simulink model "cartesian_waypoints_planner"  (R2020a)
settings: Solver=ode3  StartTime=0.0  StopTime=inf  FixedStep=0.01  RelTol=1e-3
undefined symbols (not defined in the file or in its folder): Header, Pose, TimeFromStart
libraries: robotlib x35, robotmaniplib x2, robotcorelib x1
settings Model: Creator=ROS_PO  LastModifiedBy=difra
settings OptimizationCC: EnhancedBackFolding=on  PassReuseOutputArgsAs=Individual arguments  ZeroExternalMemoryAtStartup=off  ZeroInternalMemoryAtStartup=off  MaxStackSize=64  OptimizeBlockOrder=speed  DifferentSizesBufferReuse=on  OptimizationCustomize=off  EfficientTunableParamExpr=on
settings DebuggingCC: ParameterTunabilityLossMsg=error
settings HardwareCC: ProdBitPerPointer=32  ProdBitPerSizeT=32  ProdBitPerPtrDiffT=32  ProdLargestAtomicFloat=None  ProdIntDivRoundTo=Undefined  ProdEndianess=Unspecified  ProdWordSize=32  ProdHWDeviceType=Generic->Unspecified (assume 32-bit Generic)
settings RTWCC: SystemTargetFile=ert.tlc  HardwareBoard=Robot Operating System (ROS)  TemplateMakefile=ert_default_tmf  GenerateReport=on  Toolchain=Catkin  IncludeHyperlinkInReport=on  LaunchReport=on  TargetLang=C++  GenerateTraceInfo=on  GenerateTraceReport=on  GenerateTraceReportSl=on  GenerateTraceReportSf=on  GenerateTraceReportEml=on
settings CodeAppCC: ForceParamTrailComments=on  IgnoreCustomStorageClasses=off  OperatorAnnotations=on  SimulinkDataObjDesc=on  SFDataObjDesc=on  InsertBlockDesc=on
settings ERTTargetCC: SupportContinuousTime=on  SupportVariableSizeSignals=on

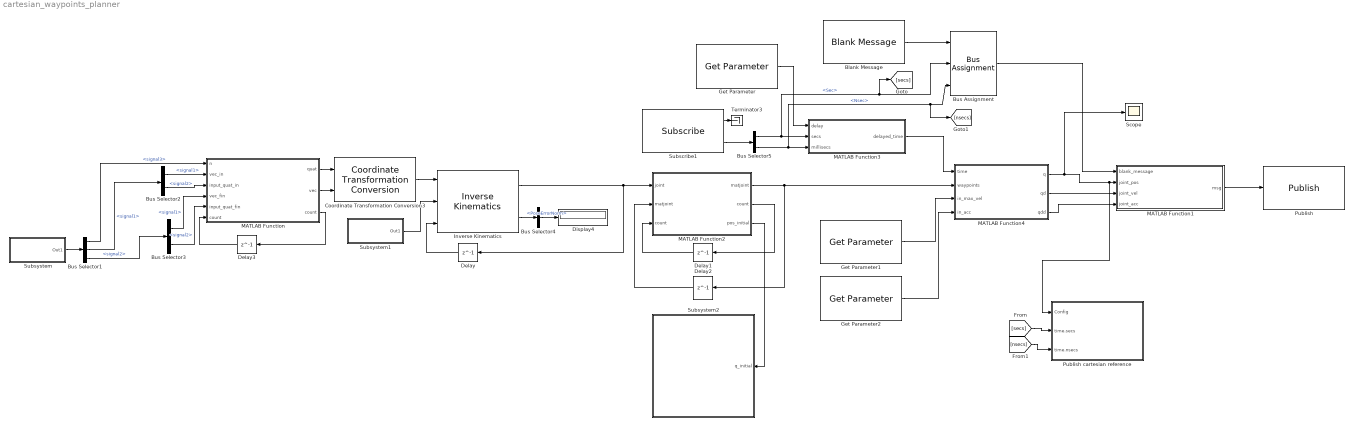
== system cartesian_waypoints_planner ==
  Blank Message : robotlib/Blank Message  messageClass=Message  entityType=trajectory_msgs/JointTrajectoryPoint  messageType=trajectory_msgs/JointTrajectoryPoint  SampleTime=-1
  Bus Assignment : BusAssignment  AssignedSignals=TimeFromStart.Sec,TimeFromStart.Nsec
  Bus Selector1 : BusSelector  OutputSignals=signal3,signal1,signal2
  Bus Selector2 : BusSelector  OutputSignals=signal1,signal2
  Bus Selector3 : BusSelector  OutputSignals=signal1,signal2
  Bus Selector4 : BusSelector  OutputSignals=PoseErrorNorm
  Bus Selector5 : BusSelector  OutputSignals=Clock_.Sec,Clock_.Nsec
  Coordinate Transformation Conversion3 : robotcorelib/Coordinate Transformation Conversion  InputRepresentation=Quaternion  InputEulerSequence=ZYX  ShowTrVecInputPort=on  OutputRepresentation=Homogeneous Transformation  OutputEulerSequence=ZYX  ShowTrVecOutputPort=on  SimulateUsing=Interpreted execution
      settings: SourceProductBaseCode=NV,RO,RR
  Delay : Delay  DelayLength=1  InitialCondition=zeros(6, 1, 1)
  Delay1 : Delay  DelayLength=1  InitialCondition=1
  Delay2 : Delay  DelayLength=1  InitialCondition=zeros(6, 20)
  Delay3 : Delay  DelayLength=1  InitialCondition=1
  Display4 : Display
  Get Parameter : robotlib/Get Parameter  ParameterSource=Specify your own  ParameterName=/start_delay  ParameterType=double  ParameterMaxArrayLength=16  ParameterInitialValue=10  SampleTime=-1  ShowErrorCodeOutput=off  ModelName=cartesian_waypoints_planner  BlockId=ParamGet_cartesian_waypoints_planner_378
      settings: SourceProductBaseCode=RR
  Get Parameter1 : robotlib/Get Parameter  ParameterSource=Specify your own  ParameterName=/max_ang_vel  ParameterType=double  ParameterMaxArrayLength=16  ParameterInitialValue=1  SampleTime=-1  ShowErrorCodeOutput=off  ModelName=cartesian_waypoints_planner  BlockId=ParamGet_cartesian_waypoints_planner_379
      settings: SourceProductBaseCode=RR
  Get Parameter2 : robotlib/Get Parameter  ParameterSource=Specify your own  ParameterName=/max_ang_acc  ParameterType=double  ParameterMaxArrayLength=16  ParameterInitialValue=0.5  SampleTime=-1  ShowErrorCodeOutput=off  ModelName=cartesian_waypoints_planner  BlockId=ParamGet_cartesian_waypoints_planner_380
      settings: SourceProductBaseCode=RR
  Inverse Kinematics : robotmaniplib/Inverse Kinematics  RigidBodyTree=robot  EndEffector=edo_link_ee  ShowInfo=on  SolverName=BFGS Gradient Projection  EnforceJointLimits=on  MaxIterations=1500  MaxTime=10  GradientTolerance=1e-7  SolutionTolerance=1e-6  StepTolerance=1e-14  ErrorChangeTolerance=1e-12  UseErrorDamping=on  DampingBias=0.0025  SimulateUsing=Interpreted execution
  MATLAB Function : MATLAB Function  TreatAsAtomicUnit=on
  MATLAB Function1 : MATLAB Function  TreatAsAtomicUnit=on
  MATLAB Function2 : MATLAB Function  TreatAsAtomicUnit=on
  MATLAB Function3 : MATLAB Function  TreatAsAtomicUnit=on
  MATLAB Function4 : MATLAB Function  TreatAsAtomicUnit=on
  Publish : robotlib/Publish  topicSource=Select from ROS network  topic=/joint_trajectory  messageType=trajectory_msgs/JointTrajectoryPoint  messageQueueLength=1
      link override SinkBlock: ROSTopic=/joint_trajectory  ROSMessageType=trajectory_msgs/JointTrajectoryPoint  SLBusName=SL_Bus_joint_trajectory_planner_JointTrajectoryPoint_y0wep  ModelName=joint_trajectory_planner  BlockId=Pub_joint_trajectory_planner_5
  Publish cartesian reference : Subsystem
  Scope : Scope
  Subscribe1 : robotlib/Subscribe  topicSource=Specify your own  topic=/clock  messageType=rosgraph_msgs/Clock  sampleTime=-1  messageQueueLength=1
  Subsystem : Subsystem
  Subsystem1 : Subsystem
  Subsystem2 : Subsystem
  Terminator3 : Terminator
  wires:
  Subsystem1/1(Out1) -> Inverse Kinematics/2
  Bus Selector4/1 -> Display4/1  "<PoseErrorNorm>"
  Inverse Kinematics/1 -> Delay/1, MATLAB Function2/1(joint)
  Inverse Kinematics/2 -> Bus Selector4/1
  Delay/1 -> Inverse Kinematics/3
  Subsystem/1(Out1) -> Bus Selector1/1
  Delay1/1 -> MATLAB Function2/3("count ")
  MATLAB Function2/2(count) -> Delay1/1
  Delay2/1 -> MATLAB Function2/2("matjoint ")
  MATLAB Function/3(count) -> Delay3/1
  Delay3/1 -> MATLAB Function/6("count ")
  MATLAB Function/1(quat) -> Coordinate Transformation Conversion3/1
  MATLAB Function/2(vec) -> Coordinate Transformation Conversion3/2
  Coordinate Transformation Conversion3/1 -> Inverse Kinematics/1
  Bus Selector2/1 -> MATLAB Function/2(vec_in)  "<signal1>"
  Bus Selector2/2 -> MATLAB Function/3(input_quat_in)  "<signal2>"
  Bus Selector3/1 -> MATLAB Function/4(vec_fin)  "<signal1>"
  Bus Selector3/2 -> MATLAB Function/5(input_quat_fin)  "<signal2>"
  Bus Selector1/3 -> Bus Selector3/1  "<signal2>"
  Bus Selector1/2 -> Bus Selector2/1  "<signal1>"
  Bus Selector1/1 -> MATLAB Function/1(n)  "<signal3>"
  MATLAB Function2/3(pos_initial) -> Subsystem2/1(q_initial)
  Subscribe1/1 -> Terminator3/1
  Get Parameter1/1 -> MATLAB Function4/3(in_max_vel)
  Bus Selector5/1 -> [secs], Bus Assignment/2, MATLAB Function3/2(secs)  "<Sec>"
  Bus Selector5/2 -> [nsecs], Bus Assignment/3, MATLAB Function3/3(millisecs)  "<Nsec>"
  Get Parameter/1 -> MATLAB Function3/1(delay)
  Subscribe1/2 -> Bus Selector5/1
  Get Parameter2/1 -> MATLAB Function4/4(in_acc)
  MATLAB Function4/2(qd) -> MATLAB Function1/3(joint_vel)
  MATLAB Function4/1(q) -> Scope/1, Publish cartesian reference/1(Config), MATLAB Function1/2(joint_pos)
  Blank Message/1 -> Bus Assignment/1
  MATLAB Function1/1(msg) -> Publish/1
  MATLAB Function4/3(qdd) -> MATLAB Function1/4(joint_acc)
  Bus Assignment/1 -> MATLAB Function1/1(blank_message)
  [nsecs] -> Publish cartesian reference/3(time.nsecs)
  [secs] -> Publish cartesian reference/2(time.secs)
  MATLAB Function3/1(delayed_time) -> MATLAB Function4/1(time)
  MATLAB Function2/1(matjoint) -> MATLAB Function4/2(waypoints), Delay2/1

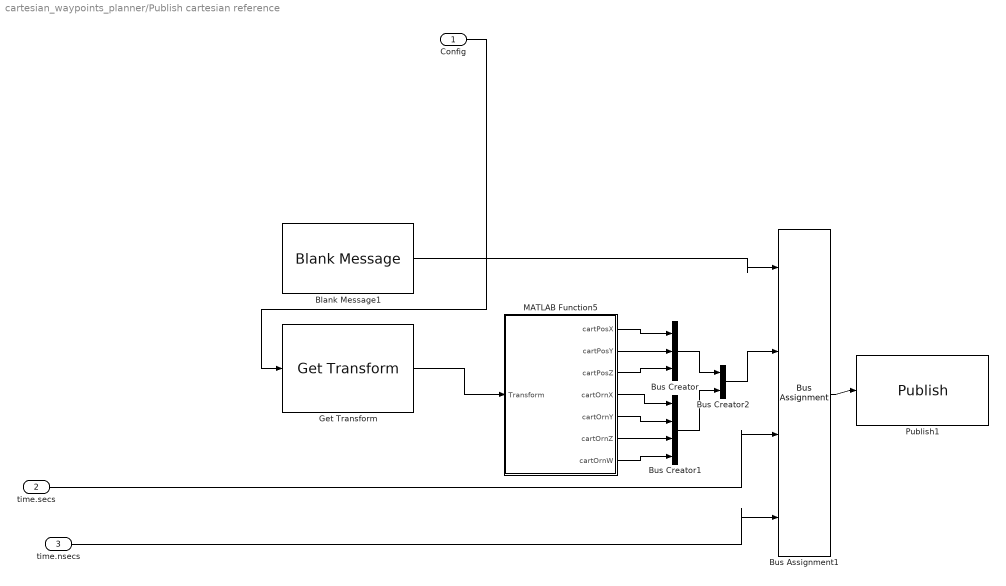
== system cartesian_waypoints_planner/Publish cartesian reference ==
  Config : Inport
  time.secs : Inport  Port=2
  time.nsecs : Inport  Port=3
  Blank Message1 : robotlib/Blank Message  messageClass=Message  entityType=geometry_msgs/PoseStamped  messageType=geometry_msgs/PoseStamped  SampleTime=inf
  Bus Assignment1 : BusAssignment  AssignedSignals=Pose,Header.Stamp.Sec,Header.Stamp.Nsec
  Bus Creator : BusCreator  Inputs=3
  Bus Creator1 : BusCreator  Inputs=4
  Bus Creator2 : BusCreator  Inputs=2
  Get Transform : robotmaniplib/Get Transform  RigidBodyTree=robot  SourceBody=edo_link_ee  TargetBody=world  SimulateUsing=Interpreted execution
  MATLAB Function5 : MATLAB Function  TreatAsAtomicUnit=on
  Publish1 : robotlib/Publish  topicSource=Specify your own  topic=/cartesian_trajectory  messageType=geometry_msgs/PoseStamped  messageQueueLength=1
  wires:
  Bus Creator1/1 -> Bus Creator2/2
  time.secs/1 -> Bus Assignment1/3
  MATLAB Function5/3(cartPosZ) -> Bus Creator/3
  MATLAB Function5/6(cartOrnZ) -> Bus Creator1/3
  time.nsecs/1 -> Bus Assignment1/4
  MATLAB Function5/5(cartOrnY) -> Bus Creator1/2
  MATLAB Function5/4(cartOrnX) -> Bus Creator1/1
  MATLAB Function5/2(cartPosY) -> Bus Creator/2
  Get Transform/1 -> MATLAB Function5/1(Transform)
  MATLAB Function5/7(cartOrnW) -> Bus Creator1/4
  Config/1 -> Get Transform/1
  Bus Creator/1 -> Bus Creator2/1
  MATLAB Function5/1(cartPosX) -> Bus Creator/1
  Bus Assignment1/1 -> Publish1/1
  Bus Creator2/1 -> Bus Assignment1/2
  Blank Message1/1 -> Bus Assignment1/1

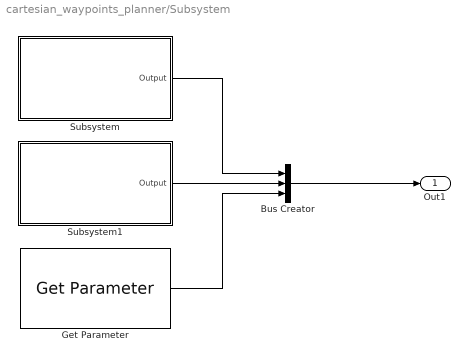
== system cartesian_waypoints_planner/Subsystem ==
  Bus Creator : BusCreator  Inputs=3
  Get Parameter : robotlib/Get Parameter  ParameterSource=Specify your own  ParameterName=/n_points  ParameterType=int32  ParameterMaxArrayLength=16  ParameterInitialValue=3  SampleTime=-1  ShowErrorCodeOutput=off  ModelName=cartesian_waypoints_planner  BlockId=ParamGet_cartesian_waypoints_planner_346
      settings: SourceProductBaseCode=RR
  Subsystem : Subsystem
  Subsystem1 : Subsystem
  Out1 : Outport
  wires:
  Bus Creator/1 -> Out1/1
  Subsystem/1(Output) -> Bus Creator/1
  Get Parameter/1 -> Bus Creator/3
  Subsystem1/1(Output) -> Bus Creator/2

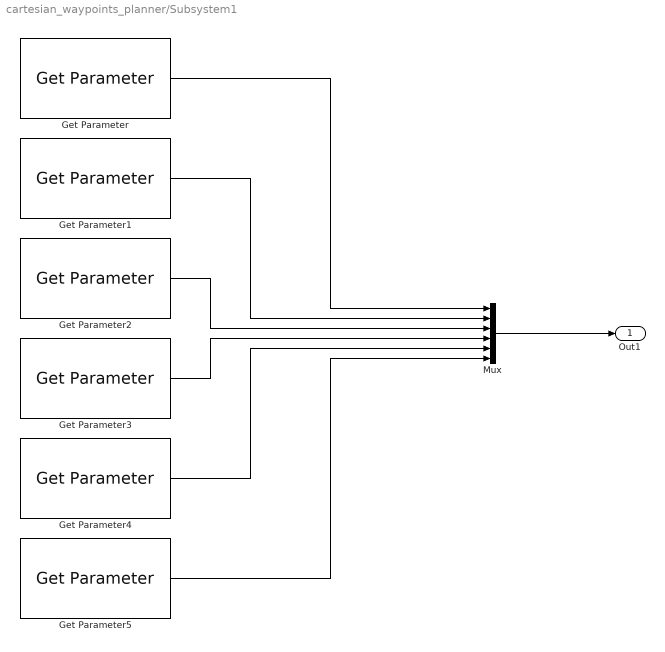
== system cartesian_waypoints_planner/Subsystem1 ==
  Get Parameter : robotlib/Get Parameter  ParameterSource=Specify your own  ParameterName=/weight_ox  ParameterType=double  ParameterMaxArrayLength=16  ParameterInitialValue=0  SampleTime=-1  ShowErrorCodeOutput=off  ModelName=cartesian_waypoints_planner  BlockId=ParamGet_cartesian_waypoints_planner_312
      settings: SourceProductBaseCode=RR
  Get Parameter1 : robotlib/Get Parameter  ParameterSource=Specify your own  ParameterName=/weight_oy  ParameterType=double  ParameterMaxArrayLength=16  ParameterInitialValue=0  SampleTime=-1  ShowErrorCodeOutput=off  ModelName=cartesian_waypoints_planner  BlockId=ParamGet_cartesian_waypoints_planner_313
      settings: SourceProductBaseCode=RR
  Get Parameter2 : robotlib/Get Parameter  ParameterSource=Specify your own  ParameterName=/weight_oz  ParameterType=double  ParameterMaxArrayLength=16  ParameterInitialValue=0  SampleTime=-1  ShowErrorCodeOutput=off  ModelName=cartesian_waypoints_planner  BlockId=ParamGet_cartesian_waypoints_planner_314
      settings: SourceProductBaseCode=RR
  Get Parameter3 : robotlib/Get Parameter  ParameterSource=Specify your own  ParameterName=/weight_px  ParameterType=double  ParameterMaxArrayLength=16  ParameterInitialValue=1  SampleTime=-1  ShowErrorCodeOutput=off  ModelName=cartesian_waypoints_planner  BlockId=ParamGet_cartesian_waypoints_planner_315
      settings: SourceProductBaseCode=RR
  Get Parameter4 : robotlib/Get Parameter  ParameterSource=Specify your own  ParameterName=/weight_py  ParameterType=double  ParameterMaxArrayLength=16  ParameterInitialValue=1  SampleTime=-1  ShowErrorCodeOutput=off  ModelName=cartesian_waypoints_planner  BlockId=ParamGet_cartesian_waypoints_planner_316
      settings: SourceProductBaseCode=RR
  Get Parameter5 : robotlib/Get Parameter  ParameterSource=Specify your own  ParameterName=/weight_pz  ParameterType=double  ParameterMaxArrayLength=16  ParameterInitialValue=1  SampleTime=-1  ShowErrorCodeOutput=off  ModelName=cartesian_waypoints_planner  BlockId=ParamGet_cartesian_waypoints_planner_317
      settings: SourceProductBaseCode=RR
  Mux : Mux  Inputs=6
  Out1 : Outport
  wires:
  Mux/1 -> Out1/1
  Get Parameter/1 -> Mux/1
  Get Parameter1/1 -> Mux/2
  Get Parameter5/1 -> Mux/6
  Get Parameter4/1 -> Mux/5
  Get Parameter3/1 -> Mux/4
  Get Parameter2/1 -> Mux/3

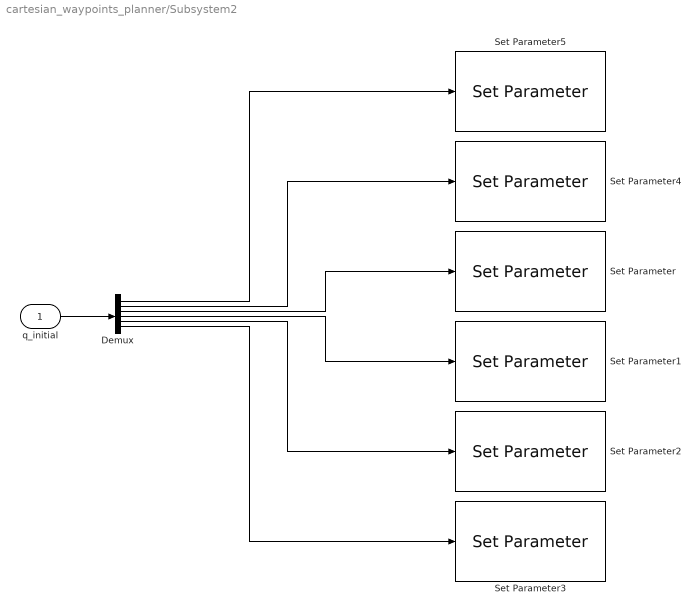
== system cartesian_waypoints_planner/Subsystem2 ==
  q_initial : Inport
  Demux : Demux  Outputs=6
  Set Parameter : robotlib/Set Parameter  ParameterSource=Specify your own  ParameterName=/q3_initial  ParameterType=double  ModelName=cartesian_waypoints_planner  BlockId=ParamSet_cartesian_waypoints_planner_364
      settings: SourceProductBaseCode=RR
  Set Parameter1 : robotlib/Set Parameter  ParameterSource=Specify your own  ParameterName=/q4_initial  ParameterType=double  ModelName=cartesian_waypoints_planner  BlockId=ParamSet_cartesian_waypoints_planner_365
      settings: SourceProductBaseCode=RR
  Set Parameter2 : robotlib/Set Parameter  ParameterSource=Specify your own  ParameterName=/q5_initial  ParameterType=double  ModelName=cartesian_waypoints_planner  BlockId=ParamSet_cartesian_waypoints_planner_366
      settings: SourceProductBaseCode=RR
  Set Parameter3 : robotlib/Set Parameter  ParameterSource=Specify your own  ParameterName=/q6_initial  ParameterType=double  ModelName=cartesian_waypoints_planner  BlockId=ParamSet_cartesian_waypoints_planner_371
      settings: SourceProductBaseCode=RR
  Set Parameter4 : robotlib/Set Parameter  ParameterSource=Specify your own  ParameterName=/q2_initial  ParameterType=double  ModelName=cartesian_waypoints_planner  BlockId=ParamSet_cartesian_waypoints_planner_372
      settings: SourceProductBaseCode=RR
  Set Parameter5 : robotlib/Set Parameter  ParameterSource=Specify your own  ParameterName=/q1_initial  ParameterType=double  ModelName=cartesian_waypoints_planner  BlockId=ParamSet_cartesian_waypoints_planner_373
      settings: SourceProductBaseCode=RR
  wires:
  q_initial/1 -> Demux/1
  Demux/1 -> Set Parameter5/1
  Demux/2 -> Set Parameter4/1
  Demux/3 -> Set Parameter/1
  Demux/4 -> Set Parameter1/1
  Demux/5 -> Set Parameter2/1
  Demux/6 -> Set Parameter3/1

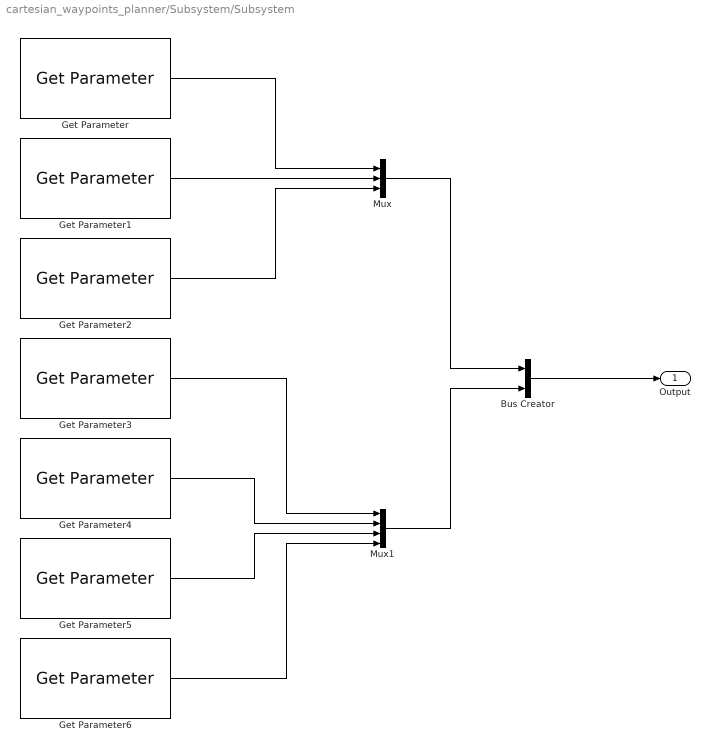
== system cartesian_waypoints_planner/Subsystem/Subsystem ==
  Bus Creator : BusCreator  Inputs=2
  Get Parameter : robotlib/Get Parameter  ParameterSource=Specify your own  ParameterName=/pi_x  ParameterType=double  ParameterMaxArrayLength=16  ParameterInitialValue=0.0  SampleTime=-1  ShowErrorCodeOutput=off  ModelName=cartesian_waypoints_planner  BlockId=ParamGet_cartesian_waypoints_planner_288
      settings: SourceProductBaseCode=RR
  Get Parameter1 : robotlib/Get Parameter  ParameterSource=Specify your own  ParameterName=/pi_y  ParameterType=double  ParameterMaxArrayLength=16  ParameterInitialValue=0.0  SampleTime=-1  ShowErrorCodeOutput=off  ModelName=cartesian_waypoints_planner  BlockId=ParamGet_cartesian_waypoints_planner_289
      settings: SourceProductBaseCode=RR
  Get Parameter2 : robotlib/Get Parameter  ParameterSource=Specify your own  ParameterName=/pi_z  ParameterType=double  ParameterMaxArrayLength=16  ParameterInitialValue=0.99  SampleTime=-1  ShowErrorCodeOutput=off  ModelName=cartesian_waypoints_planner  BlockId=ParamGet_cartesian_waypoints_planner_290
      settings: SourceProductBaseCode=RR
  Get Parameter3 : robotlib/Get Parameter  ParameterSource=Specify your own  ParameterName=/oi_x  ParameterType=double  ParameterMaxArrayLength=16  ParameterInitialValue=0  SampleTime=-1  ShowErrorCodeOutput=off  ModelName=cartesian_waypoints_planner  BlockId=ParamGet_cartesian_waypoints_planner_291
      settings: SourceProductBaseCode=RR
  Get Parameter4 : robotlib/Get Parameter  ParameterSource=Specify your own  ParameterName=/oi_y  ParameterType=double  ParameterMaxArrayLength=16  ParameterInitialValue=0.0  SampleTime=-1  ShowErrorCodeOutput=off  ModelName=cartesian_waypoints_planner  BlockId=ParamGet_cartesian_waypoints_planner_292
      settings: SourceProductBaseCode=RR
  Get Parameter5 : robotlib/Get Parameter  ParameterSource=Specify your own  ParameterName=/oi_z  ParameterType=double  ParameterMaxArrayLength=16  ParameterInitialValue=0.0  SampleTime=-1  ShowErrorCodeOutput=off  ModelName=cartesian_waypoints_planner  BlockId=ParamGet_cartesian_waypoints_planner_293
      settings: SourceProductBaseCode=RR
  Get Parameter6 : robotlib/Get Parameter  ParameterSource=Specify your own  ParameterName=/oi_w  ParameterType=double  ParameterMaxArrayLength=16  ParameterInitialValue=1  SampleTime=-1  ShowErrorCodeOutput=off  ModelName=cartesian_waypoints_planner  BlockId=ParamGet_cartesian_waypoints_planner_294
      settings: SourceProductBaseCode=RR
  Mux : Mux  Inputs=3
  Mux1 : Mux
  Output : Outport
  wires:
  Mux/1 -> Bus Creator/1
  Get Parameter/1 -> Mux/1
  Get Parameter1/1 -> Mux/2
  Get Parameter2/1 -> Mux/3
  Get Parameter3/1 -> Mux1/1
  Get Parameter4/1 -> Mux1/2
  Get Parameter5/1 -> Mux1/3
  Get Parameter6/1 -> Mux1/4
  Mux1/1 -> Bus Creator/2
  Bus Creator/1 -> Output/1

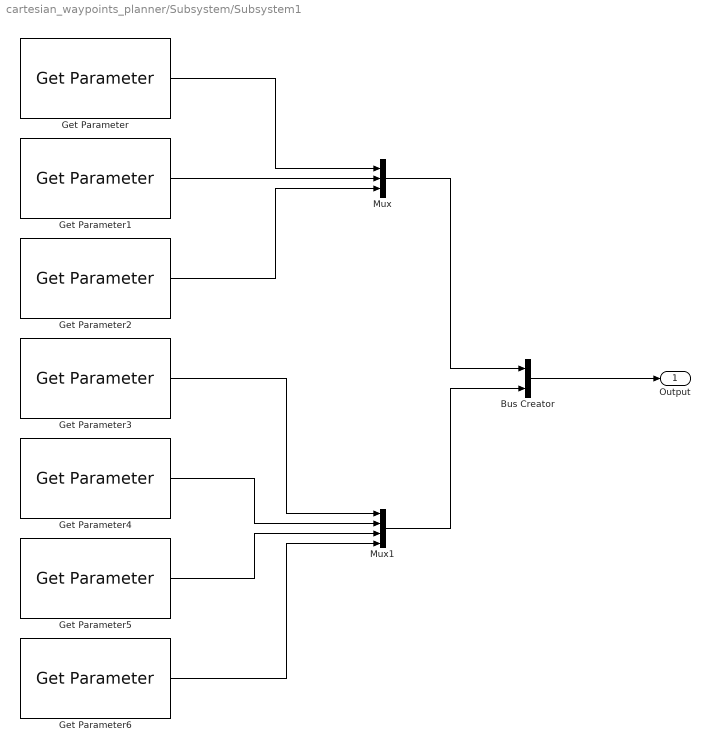
== system cartesian_waypoints_planner/Subsystem/Subsystem1 ==
  Bus Creator : BusCreator  Inputs=2
  Get Parameter : robotlib/Get Parameter  ParameterSource=Specify your own  ParameterName=/pf_x  ParameterType=double  ParameterMaxArrayLength=16  ParameterInitialValue=0.3  SampleTime=-1  ShowErrorCodeOutput=off  ModelName=cartesian_waypoints_planner  BlockId=ParamGet_cartesian_waypoints_planner_300
      settings: SourceProductBaseCode=RR
  Get Parameter1 : robotlib/Get Parameter  ParameterSource=Specify your own  ParameterName=/pf_y  ParameterType=double  ParameterMaxArrayLength=16  ParameterInitialValue=0.3  SampleTime=-1  ShowErrorCodeOutput=off  ModelName=cartesian_waypoints_planner  BlockId=ParamGet_cartesian_waypoints_planner_301
      settings: SourceProductBaseCode=RR
  Get Parameter2 : robotlib/Get Parameter  ParameterSource=Specify your own  ParameterName=/pf_z  ParameterType=double  ParameterMaxArrayLength=16  ParameterInitialValue=0.3  SampleTime=-1  ShowErrorCodeOutput=off  ModelName=cartesian_waypoints_planner  BlockId=ParamGet_cartesian_waypoints_planner_302
      settings: SourceProductBaseCode=RR
  Get Parameter3 : robotlib/Get Parameter  ParameterSource=Specify your own  ParameterName=/of_x  ParameterType=double  ParameterMaxArrayLength=16  ParameterInitialValue=0.39  SampleTime=-1  ShowErrorCodeOutput=off  ModelName=cartesian_waypoints_planner  BlockId=ParamGet_cartesian_waypoints_planner_303
      settings: SourceProductBaseCode=RR
  Get Parameter4 : robotlib/Get Parameter  ParameterSource=Specify your own  ParameterName=/of_y  ParameterType=double  ParameterMaxArrayLength=16  ParameterInitialValue=0.89  SampleTime=-1  ShowErrorCodeOutput=off  ModelName=cartesian_waypoints_planner  BlockId=ParamGet_cartesian_waypoints_planner_304
      settings: SourceProductBaseCode=RR
  Get Parameter5 : robotlib/Get Parameter  ParameterSource=Specify your own  ParameterName=/of_z  ParameterType=double  ParameterMaxArrayLength=16  ParameterInitialValue=0.2  SampleTime=-1  ShowErrorCodeOutput=off  ModelName=cartesian_waypoints_planner  BlockId=ParamGet_cartesian_waypoints_planner_305
      settings: SourceProductBaseCode=RR
  Get Parameter6 : robotlib/Get Parameter  ParameterSource=Specify your own  ParameterName=/of_w  ParameterType=double  ParameterMaxArrayLength=16  ParameterInitialValue=-0.12  SampleTime=-1  ShowErrorCodeOutput=off  ModelName=cartesian_waypoints_planner  BlockId=ParamGet_cartesian_waypoints_planner_306
      settings: SourceProductBaseCode=RR
  Mux : Mux  Inputs=3
  Mux1 : Mux
  Output : Outport
  wires:
  Mux/1 -> Bus Creator/1
  Get Parameter/1 -> Mux/1
  Get Parameter1/1 -> Mux/2
  Get Parameter2/1 -> Mux/3
  Get Parameter3/1 -> Mux1/1
  Get Parameter4/1 -> Mux1/2
  Get Parameter5/1 -> Mux1/3
  Get Parameter6/1 -> Mux1/4
  Mux1/1 -> Bus Creator/2
  Bus Creator/1 -> Output/1

== matlab function cartesian_waypoints_planner/MATLAB Function ==
  data: n input; quat output; vec_in input; vec output; input_quat_in input; vec_fin input; input_quat_fin input; count input; count output
function [quat, vec, count] = fcn(n, vec_in, input_quat_in, vec_fin, input_quat_fin, count)

    if n > 20
        n = int32(20);
    end

    quat_in = quaternion(transpose(input_quat_in));
    quat_fin = quaternion(transpose(input_quat_fin));

    quater = quaternion(zeros(1, 4));
    vec = zeros(3, 1);

    if count <= 1
        vec = vec_in;
        quater = quat_in;
    elseif count < n
        vec = (vec_fin - vec_in) / double(n) * count + vec_in;
        quater = slerp(quat_in, quat_fin, count / double(n));
    elseif count >= n
        vec = vec_fin;
        quater = quat_fin;
    end

    quat = transpose(compact(quater));

    count = count + 1;

== matlab function cartesian_waypoints_planner/MATLAB Function1 ==
  data: blank_message input; joint_pos input; msg output Bus: SL_Bus_cartesian_waypoints_plann_JointTrajectoryPoint_rocwzq; joint_vel input; joint_acc input
function msg = assign_trajectory(blank_message, joint_pos, joint_vel, joint_acc)

    msg = blank_message;
    numJoints = length(joint_vel);
    msg.Velocities_SL_Info.CurrentLength = uint32(numJoints);
    msg.Velocities(1:numJoints) = joint_vel;
    msg.Positions_SL_Info.CurrentLength = uint32(numJoints);
    msg.Positions(1:numJoints) = joint_pos;
    msg.Accelerations_SL_Info.CurrentLength = uint32(numJoints);
    msg.Accelerations(1:numJoints) = joint_acc;

== matlab function cartesian_waypoints_planner/MATLAB Function3 ==
  data: delay input; secs input; millisecs input; delayed_time output
function delayed_time = get_time(delay, secs, millisecs)

    time = secs + millisecs / 1e9;
    delayed_time = time - delay;
    
    if delayed_time < 0
        delayed_time = 0;
    end

== matlab function cartesian_waypoints_planner/MATLAB Function4 ==
  data: time input; q output; waypoints input; in_max_vel input; in_acc input; qd output; qdd output
function [q, qd, qdd] = fcn(time, waypoints, in_max_vel, in_acc)

    [rows, columns] = size(waypoints);

    q = waypoints(:, 1);
    qd = zeros(rows, 1);
    qdd = zeros(rows, 1);

    if time < 0
        time = 0;
    end

    if length(in_max_vel) == 1
        max_vel = in_max_vel * ones(rows, 1);
    else
        max_vel = in_max_vel;
    end

    if length(in_acc) == 1
        acc = in_acc * ones(rows, 1);
    else
        acc = in_acc;
    end

    signes = zeros(rows, columns-1);
    t = zeros(rows, columns-1, 3);
    d_t = zeros(rows);
    steps = ones(rows);

    for i=1:rows

        t_up = max_vel(i) / acc(i);
        t1 = time;

        for j=1:columns-1

            dist = waypoints(i, j+1) - waypoints(i, j);
            signes(i, j) = sign(dist);

            if abs(dist) < t_up * max_vel(i)
                act_t_up = sqrt(abs(dist)/acc(i));
                t(i, j, 2) = 0;
                t(i, j, 1) = act_t_up;
                t(i, j, 3) = act_t_up;
            else
                t(i, j, 1) = t_up;
                t(i, j, 3) = t_up;
                t(i, j, 2) = (abs(dist) - t_up * max_vel(i)) / max_vel(i);
            end

            if t1 - t(i, j, 1) - t(i, j, 2) - t(i, j, 3) >= 0
                steps(i) = steps(i) + 1;
                d_t(i) = d_t(i) + t(i, j, 1) + t(i, j, 2) + t(i, j, 3);
                t1 = t1 - t(i, j, 1) - t(i, j, 2) - t(i, j, 3);
            else
                break;
            end

        end

    end

    for i=1:rows

        t1 = time - d_t(i);
        j = steps(i);
        q(i) = waypoints(i, j);
        
        if j == columns
            q(i) = waypoints(i, j);
            qd(i) = 0;
            qdd(i) = 0;
            continue;
        end
        
        if t1 <= 0
            q(i) = waypoints(i, j);
            qd(i) = 0;
            qdd(i) = 0;
        elseif t1 - t(i, j, 1)  < 0
            q(i) = q(i) + 1/2 * acc(i) * t1^2 * signes(i, j);
            qd(i) = acc(i) * t1 * signes(i, j);
            qdd(i) = acc(i) * signes(i, j);
        elseif t1 - t(i, j, 1) - t(i, j, 2) < 0
            q(i) = q(i) + max_vel(i, j) * (t1 - t(i, j, 1) / 2) * signes(i, j);
            qd(i) = max_vel(i, j) * signes(i, j);
            qdd(i) = 0;
        elseif t1 - t(i, j, 1) - t(i, j, 2) - t(i, j, 3) < 0
            q(i) = waypoints(i, j+1) - 1/2 * acc(i) * (t(i, j, 1) + t(i, j, 2) + t(i, j, 3) - t1) ^ 2 * signes(i, j);
            qd(i) =  acc(i) * (t(i, j, 1) + t(i, j, 2) + t(i, j, 3) - t1) * signes(i, j);
            qdd(i) = - acc(i) * signes(i, j);
        else
            q(i) = waypoints(i, j);
            qd(i) = 0;
            qdd(i) = 0;
        end


    end

== matlab function cartesian_waypoints_planner/MATLAB Function2 ==
  data: matjoint output; joint input; matjoint input; count output; count input; pos_initial output
function [matjoint, count, pos_initial] = fcn(joint, matjoint, count)

% matrice di waypoints 6x20

if count >= 1 && count <= 20
    matjoint(1:6, count) = joint;
end

pos_initial=matjoint(1:6,1);

count = count + 1;

== matlab function cartesian_waypoints_planner/Publish cartesian reference/MATLAB Function5 ==
  data: Transform input; cartPosX output; cartPosY output; cartPosZ output; cartOrnX output; cartOrnY output; cartOrnZ output; cartOrnW output
function [cartPosX, cartPosY, cartPosZ, cartOrnX, cartOrnY, cartOrnZ, cartOrnW] = calculate_cartesian_state(Transform)

    cartPos = Transform(1:3, 4);
    cartOrn = rotm2quat(Transform(1:3, 1:3));
    
    cartPosX = cartPos(1);
    cartPosY = cartPos(2);
    cartPosZ = cartPos(3);
    
    cartOrnX = cartOrn(1);
    cartOrnY = cartOrn(2);
    cartOrnZ = cartOrn(3);
    cartOrnW = cartOrn(4);
